simulink model "singular2quasiOEs"  (R2023a)
settings: Solver=ode4  StartTime=0.0  StopTime=10.0  FixedStep=dt  RelTol=1e-3
settings Model: Creator=hugobuurmeijer  LastModifiedBy=ndelurgio

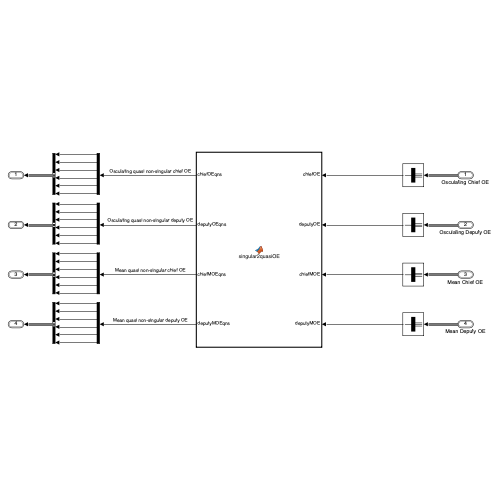
[thumbnail: Simulink's stored preview of the top-level diagram]
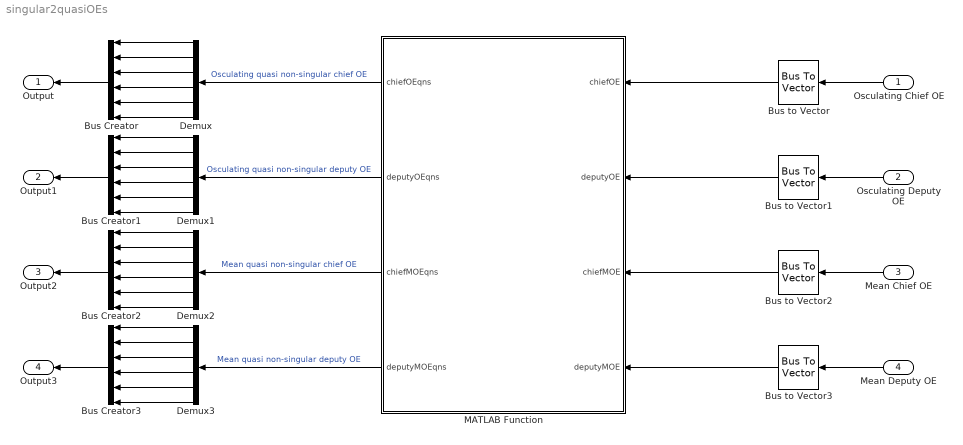
== system singular2quasiOEs ==
  Osculating Chief OE : Inport  OutDataTypeStr=Bus: osculatingOrbitElements
  Osculating Deputy OE : Inport  Port=2  OutDataTypeStr=Bus: osculatingOrbitElements
  Mean Chief OE : Inport  Port=3  OutDataTypeStr=Bus: meanOrbitElements
  Mean Deputy OE : Inport  Port=4  OutDataTypeStr=Bus: meanOrbitElements
  Bus Creator : BusCreator  Inputs=6  OutDataTypeStr=Bus: osculatingOrbitElementsQNS
  Bus Creator1 : BusCreator  Inputs=6  OutDataTypeStr=Bus: osculatingOrbitElementsQNS
  Bus Creator2 : BusCreator  Inputs=6  OutDataTypeStr=Bus: meanOrbitElementsQNS
  Bus Creator3 : BusCreator  Inputs=6  OutDataTypeStr=Bus: meanOrbitElementsQNS
  Bus to Vector{,1..3} (4 alike) : BusToVector
  Demux{,1..3} (4 alike) : Demux  Outputs=6
  MATLAB Function : MATLAB Function  TreatAsAtomicUnit=on
  Output : Outport  OutDataTypeStr=Bus: osculatingOrbitElementsQNS
  Output1 : Outport  Port=2  OutDataTypeStr=Bus: osculatingOrbitElementsQNS
  Output2 : Outport  Port=3  OutDataTypeStr=Bus: meanOrbitElementsQNS
  Output3 : Outport  Port=4  OutDataTypeStr=Bus: meanOrbitElementsQNS
  wires:
  Osculating Deputy OE/1 -> Bus to Vector1/1
  Bus to Vector3/1 -> MATLAB Function/4(deputyMOE)
  Mean Deputy OE/1 -> Bus to Vector3/1
  Bus to Vector/1 -> MATLAB Function/1(chiefOE)
  Bus to Vector1/1 -> MATLAB Function/2(deputyOE)
  Mean Chief OE/1 -> Bus to Vector2/1
  Osculating Chief OE/1 -> Bus to Vector/1
  Bus to Vector2/1 -> MATLAB Function/3(chiefMOE)
  Demux/6 -> Bus Creator/6
  Demux/2 -> Bus Creator/2
  Bus Creator/1 -> Output/1
  Demux/4 -> Bus Creator/4
  Demux/3 -> Bus Creator/3
  Demux/5 -> Bus Creator/5
  Demux/1 -> Bus Creator/1
  MATLAB Function/1(chiefOEqns) -> Demux/1  "Osculating quasi non-singular chief OE"
  Bus Creator1/1 -> Output1/1
  Demux1/6 -> Bus Creator1/6
  Demux1/4 -> Bus Creator1/4
  Demux1/3 -> Bus Creator1/3
  Demux1/2 -> Bus Creator1/2
  Demux1/1 -> Bus Creator1/1
  Demux1/5 -> Bus Creator1/5
  MATLAB Function/2(deputyOEqns) -> Demux1/1  "Osculating quasi non-singular deputy OE"
  Demux2/6 -> Bus Creator2/6
  Bus Creator2/1 -> Output2/1
  Demux2/3 -> Bus Creator2/3
  Demux2/5 -> Bus Creator2/5
  MATLAB Function/3(chiefMOEqns) -> Demux2/1  "Mean quasi non-singular chief OE"
  Demux2/2 -> Bus Creator2/2
  Demux2/4 -> Bus Creator2/4
  Demux3/6 -> Bus Creator3/6
  Bus Creator3/1 -> Output3/1
  Demux3/3 -> Bus Creator3/3
  Demux3/5 -> Bus Creator3/5
  MATLAB Function/4(deputyMOEqns) -> Demux3/1  "Mean quasi non-singular deputy OE"
  Demux3/2 -> Bus Creator3/2
  Demux3/4 -> Bus Creator3/4
  Demux2/1 -> Bus Creator2/1
  Demux3/1 -> Bus Creator3/1

== matlab function singular2quasiOEs/MATLAB Function ==
  data: chiefOEqns output; deputyOEqns output; chiefMOEqns output; deputyMOEqns output; chiefOE input; deputyOE input; chiefMOE input; deputyMOE input
function [chiefOEqns, deputyOEqns, chiefMOEqns, deputyMOEqns] = singular2quasiOE(chiefOE, deputyOE, chiefMOE, deputyMOE)

chiefOEqns = singular2quasiOE(chiefOE);
deputyOEqns = singular2quasiOE(deputyOE);
chiefMOEqns = singular2quasiOE(chiefMOE);
deputyMOEqns = singular2quasiOE(deputyMOE);

end
